simulink model "convolution"  (Simulink 8.3)
settings: Solver=FixedStepDiscrete  StartTime=0.0  StopTime=0.01  FixedStep=1e-5  MaxStep=1e-4  RelTol=1e-3
settings Model: Creator=Administrator  LastModifiedBy=Administrator
settings SolverCC: ShapePreserveControl=EnableAll
settings DataIOCC: SignalLoggingSaveFormat=Dataset
settings DebuggingCC: AlgebraicLoopMsg=none  UnderspecifiedInitializationDetection=Simplified  SolverPrmCheckMsg=none  StateNameClashWarn=none
settings GRTTargetCC: CombineOutputUpdateFcns=on  GRTInterface=off

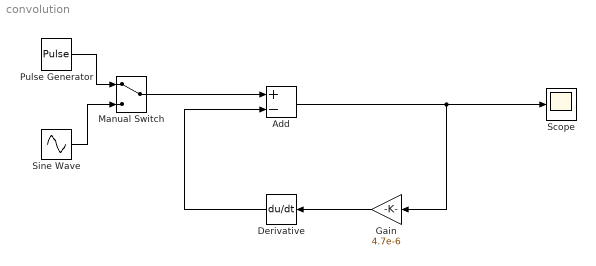
== system convolution ==
  Add : Sum  Inputs=+-
  Derivative : Derivative
  Gain : Gain  Gain=4.7e-6
  Manual Switch : ManualSwitch
  Pulse Generator : DiscretePulseGenerator  PulseType=Time based  Amplitude=5  Period=2e-4  PulseWidth=50
  Scope : Scope
  Sine Wave : Sin  Amplitude=5  Frequency=2*pi*5000  SampleTime=0
  wires:
  Derivative/1 -> Add/2
  Gain/1 -> Derivative/1
  Add/1 -> Gain/1, Scope/1
  Manual Switch/1 -> Add/1
  Pulse Generator/1 -> Manual Switch/1
  Sine Wave/1 -> Manual Switch/2
